simulink model "npc_controller"  (R2022a)
settings: Solver=FixedStepDiscrete  StartTime=0.0  StopTime=20  RelTol=1e-3  EnableMultiTasking=on
undefined symbols (not defined in the file): CAN_O_INT, CANA_BASE, Down, GPTRIP1SEL, GPTRIP2SEL, GPTRIP3SEL, Tsw, TZ1, TZ2, TZ3, Up
libraries: simulink x147, hdlsllib x90, c2802xlib x34, c2837xDlib x20, c280xlib x12, canmsglib x9, c2838xlib x8, idelinklib_common x3, c2806xlib x2, slpidlib x2, c28004xlib x2, c281xlib x2
(part 8 of 42)

== system npc_controller/CONTROL/STATE-MACHINE/CPU_CONTROL_750_A2_precharge_pfc_ok2_OL SS1/disablePwm ==
  note: /*Force PWM to LOW*/
      | EPwm2Regs.AQCSFRC.bit.CSFA = (uint16_T)(0b01);
      | EPwm2Regs.AQCSFRC.bit.CSFB = (uint16_T)(0b01);
      | EPwm7Regs.AQCSFRC.bit.CSFA = (uint16_T)(0b01);
      | EPwm7Regs.AQCSFRC.bit.CSFB = (uint16_T)(0b01);
      | EPwm8Regs.AQCSFRC.bit.CSFA = (uint16_T)(0b01);
      | EPwm8Regs.AQCSFRC.bit.CSFB = (uint16_T)(0b01);
      | EPwm9Regs.AQCSFRC.bit.CSFA = (uint16_T)(0b01);
      | EPwm9Regs.AQCSFRC.bit.CSFB = (uint16_T)(0b01);
      | EPwm10Regs.AQCSFRC.bit.CSFA = (uint16_T)(0b01);
      | EPwm10Regs.AQCSFRC.bit.CSFB = (uint16_T)(0b01);
      | EPwm11Regs.AQCSFRC.bit.CSFA = (uint16_T)(0b01);
      | EPwm11Regs.AQCSFRC.bit.CSFB = (uint16_T)(0b01);
  note: Note:
      | AQCSFRC
      | 0b00 - disables forced PWM
      | 0b01 - forces PWM to LOW
      | 0b10 - forces PWM to  HIGH
  f : TriggerPort  TriggerType=function-call  VariantControl=(inherit)
      settings: CopyFcn=Stateflow.SLINSF.SimulinkMan.removeBlockPreDeleteFcn  PreDeleteFcn=Stateflow.SLINSF.SimulinkMan.unsafePredeleteFcn
  System Outputs : Subsystem  mask(System Outputs){ShowInLibBrowser=0}
      mask prompts: ShowInLibBrowser "Simulink:masks:CustCodeMaskParam1_MP"
      settings: CopyFcn=cccopyfcn(gcb)  OpenFcn=ccopenfcn('System Outputs Function')
      mask Help: eval('feval(''rtwprivate'',''rtwhelpview'',''rtw_sys_outputs_block'')');
      mask Display: disp('System\nOutputs');

== system npc_controller/CONTROL/STATE-MACHINE/CPU_CONTROL_750_A2_precharge_pfc_ok2_OL SS1/enDigCmpMode ==
  note: Note:
      | TZCCTL
      | 0b00 - High impedance
      | 0b01 - Force to HIGH
      | 0b10 - Force to LOW
      | 0b11 - Do nothing
  note: /*Configure TZCTL*/
      | //TZCTL configures TZ action of a DCxEVTy event
      | //0b00=HI-Z, 0b01=HI, 0b10=LO, 0b11=DN
      | EALLOW;
      | EPwm2Regs.TZCTL.bit.DCAEVT1 = 0b10;
      | EPwm2Regs.TZCTL.bit.DCAEVT2 = 0b01;
      | EPwm7Regs.TZCTL.bit.DCAEVT1 = 0b10;
      | EPwm7Regs.TZCTL.bit.DCAEVT2 = 0b01;
      |
      | EPwm8Regs.TZCTL.bit.DCBEVT1 = 0b10;
      | EPwm8Regs.TZCTL.bit.DCBEVT2 = 0b01;
      | EPwm9Regs.TZCTL.bit.DCAEVT1 = 0b10;
      | EPwm9Regs.TZCTL.bit.DCAEVT2 = 0b01;
      |
      | EPwm10Regs.TZCTL.bit.DCBEVT1 = 0b10;
      | EPwm10Regs.TZCTL.bit.DCBEVT2 = 0b01;
      | EPwm11Regs.TZCTL.bit.DCAEVT1 = 0b10;
      | EPwm11Regs.TZCTL.bit.DCAEVT2 = 0b01;
      | EDIS;
  f : TriggerPort  TriggerType=function-call  VariantControl=(inherit)
      settings: CopyFcn=Stateflow.SLINSF.SimulinkMan.removeBlockPreDeleteFcn  PreDeleteFcn=Stateflow.SLINSF.SimulinkMan.unsafePredeleteFcn
  System Outputs2 : Subsystem  mask(System Outputs){ShowInLibBrowser=0}
      mask prompts: ShowInLibBrowser "Simulink:masks:CustCodeMaskParam1_MP"
      settings: CopyFcn=cccopyfcn(gcb)  OpenFcn=ccopenfcn('System Outputs Function')
      mask Help: eval('feval(''rtwprivate'',''rtwhelpview'',''rtw_sys_outputs_block'')');
      mask Display: disp('System\nOutputs');

== system npc_controller/CONTROL/STATE-MACHINE/CPU_CONTROL_750_A2_precharge_pfc_ok2_OL SS1/updateCalib ==
  note: Note: 50 cycles of 50Hz vac
  cnt_calib : Inport  OutDataTypeStr=uint16  PortDimensions=1
  van : Inport  Port=2  OutDataTypeStr=single  PortDimensions=1
  vbn : Inport  Port=3  OutDataTypeStr=single  PortDimensions=1
  vcn : Inport  Port=4  OutDataTypeStr=single  PortDimensions=1
  ia : Inport  Port=5  OutDataTypeStr=single  PortDimensions=1
  ib : Inport  Port=6  OutDataTypeStr=single  PortDimensions=1
  ic : Inport  Port=7  OutDataTypeStr=single  PortDimensions=1
  f : TriggerPort  TriggerType=function-call  VariantControl=(inherit)
      settings: CopyFcn=Stateflow.SLINSF.SimulinkMan.removeBlockPreDeleteFcn  PreDeleteFcn=Stateflow.SLINSF.SimulinkMan.unsafePredeleteFcn
  If : If  IfExpression=u1 > 65000
  If1 : If  Commented=on  IfExpression=u1 > 13000
  Merge : Merge
  Scope : Scope  Commented=on
  cnt : Subsystem  TreatAsAtomicUnit=on
  done : Subsystem  TreatAsAtomicUnit=on
  calib_ok : Outport
  wires:
  cnt_calib/1 -> If/1, cnt/1(cnt_calib)
  cnt/1(calib_ok) -> Merge/2
  done/1(calib_ok) -> Merge/1
  If/1 -> done/Action
  If/2 -> cnt/Action
  Merge/1 -> calib_ok/1, Scope/1
  van/1 -> cnt/2(van)
  vbn/1 -> cnt/3(vbn)
  vcn/1 -> cnt/4(vcn)
  ia/1 -> cnt/5(ia)
  ib/1 -> cnt/6(ib)
  ic/1 -> cnt/7(ic)

== system npc_controller/CONTROL/STATE-MACHINE/CPU_CONTROL_750_A2_precharge_pfc_ok2_OL SS1/updatePll3p ==
  van : Inport  OutDataTypeStr=double  PortDimensions=1
  vbn : Inport  Port=2  OutDataTypeStr=double  PortDimensions=1
  vcn : Inport  Port=3  OutDataTypeStr=double  PortDimensions=1
  f : TriggerPort  TriggerType=function-call  VariantControl=(inherit)
      settings: CopyFcn=Stateflow.SLINSF.SimulinkMan.removeBlockPreDeleteFcn  PreDeleteFcn=Stateflow.SLINSF.SimulinkMan.unsafePredeleteFcn
  Mux : Mux  Inputs=3
  PLL : Subsystem  TreatAsAtomicUnit=on
      settings: RTWFcnNameOpts=Use subsystem name
  Scope : Scope  NumInputPorts=4
  theta : Outport
  wires:
  PLL/1(theta) -> Scope/4, theta/1
  van/1 -> Scope/1, Mux/1
  vcn/1 -> Scope/3, Mux/3
  vbn/1 -> Scope/2, Mux/2
  Mux/1 -> PLL/1(abc)

== system npc_controller/CONTROL/STATE-MACHINE/CPU_CONTROL_750_A2_precharge_pfc_ok2_OL SS1/updateSequencePhA ==
  note: Note:
      | Vmid         C2
      | Vbulk        A5
      |
      | Va            A2/B6
      | Vb            B0
      | Vc            C0
      |
      | Ia             A3
      | Ib             A10/B1, C10
      | Ic             C1
  note: Notes:
      | vac_adc = vac_actual*0.00264706+1.65
      | iac_adc = iac_actual*0.02+1.65
      | vbulk_adc = vbulk_actual*3.49e-3
      | vmid_adc = vmid_acutal*3.49e-3
  vxn : Inport
  ix : Inport  Port=2
  f : TriggerPort  TriggerType=function-call  VariantControl=(inherit)
      settings: CopyFcn=Stateflow.SLINSF.SimulinkMan.removeBlockPreDeleteFcn  PreDeleteFcn=Stateflow.SLINSF.SimulinkMan.unsafePredeleteFcn
  Cast To Single : DataTypeConversion  Commented=on  OutDataTypeStr=single  SaturateOnIntegerOverflow=off  RndMeth=Floor
  Cast To Single1 : DataTypeConversion  Commented=on  OutDataTypeStr=single  SaturateOnIntegerOverflow=off  RndMeth=Floor
  From5 : From  Commented=on  GotoTag=vxn
  From6 : From  Commented=on  GotoTag=pol_vxn
  From7 : From  Commented=on  GotoTag=ix
  From8 : From  Commented=on  GotoTag=pol_ix
  Function-Call Generator : simulink/Ports & Subsystems/Function-Call Generator  sample_time=-1  numberOfIterations=1  DisallowWideOutput=off
  Function-Call Split : FunctionCallSplit  NumOutputPorts=2
  Function-Call Split2 : FunctionCallSplit  NumOutputPorts=2
  Gain2 : Gain  Commented=on  Gain=200
  Gain3 : Gain  Commented=on  Gain=200
  Mux : Mux  Commented=on  Inputs=2
  Mux1 : Mux  Commented=on  Inputs=2
  Scope : Scope  Commented=on  NumInputPorts=3
  pol_final1 : Subsystem  Commented=on
  pol_ix1 : Subsystem  Commented=on
  pol_vxn1 : Subsystem
  vx_seq : Outport
  wires:
  vxn/1 -> [vxn]
  Function-Call Split/2 -> pol_final1/Trigger
  Function-Call Split2/1 -> pol_vxn1/Trigger
  Function-Call Split/1 -> pol_ix1/Trigger
  Function-Call Generator/1 -> Function-Call Split2/1
  Function-Call Split2/2 -> Function-Call Split/1
  [vxn] -> pol_vxn1/1(vxn)
  [ix] -> pol_ix1/1(ix)
  pol_ix1/1(pol_ix) -> [pol_ix]
  [pol_vxn] -> pol_final1/1(vxn)
  [pol_ix] -> pol_final1/2(ix)
  pol_final1/1(pol) -> Scope/3
  Mux/1 -> Scope/1
  Mux1/1 -> Scope/2
  From6/1 -> Cast To Single/1
  From8/1 -> Cast To Single1/1
  Cast To Single/1 -> Gain2/1
  ix/1 -> [ix]
  From5/1 -> Mux/1
  From7/1 -> Mux1/1
  Gain2/1 -> Mux/2
  Cast To Single1/1 -> Gain3/1
  Gain3/1 -> Mux1/2
  [pol_vxn] -> vx_seq/1
  pol_vxn1/1(pol_vxn) -> [pol_vxn]

== system npc_controller/CONTROL/STATE-MACHINE/CPU_CONTROL_750_A2_precharge_pfc_ok2_OL SS1/updateSequencePhB ==
  note: Note:
      | Vmid         C2
      | Vbulk        A5
      |
      | Va            A2/B6
      | Vb            B0
      | Vc            C0
      |
      | Ia             A3
      | Ib             A10/B1, C10
      | Ic             C1
  note: Notes:
      | vac_adc = vac_actual*0.00264706+1.65
      | iac_adc = iac_actual*0.02+1.65
      | vbulk_adc = vbulk_actual*3.49e-3
      | vmid_adc = vmid_acutal*3.49e-3
  note: Note:
      |
      | Function PWM # GPIO # LAUNCHPAD PIN #
      |
      | Synci EPWM1A GPIO0 J4.40
      | EPWM1B GPIO1 J4.39
      |
      | ORPS EPMW2A GPIO2 J4.38
      | EPWM2B GPIO3 J4.37
      |
      | RELAY EPWM3A GPIO4 J4.36
      |
      | TZ GPIO62 XX
      |
      | a_s1 EPWM6A GPIO10 J8.76
      | a_s2 EPWM7B GPIO13 XX
      | a_s3 EPWM6B GPIO11 J8.75
      | a_s4 EPWM7A GPIO12 XX
      |
      | b_s1 EPWM8B GPIO15 J8.73
      | b_s2 EPWM9B GPIO17 XX
      | b_s3 EPWM8A GPIO14 J8.74
      | b_s4 EPWM9A GPIO16 J4.33
      |
      | c_s1 EPWM10B GPIO19 J1.3
      | c_s2 EPWM11B GPIO21 XX
      | c_s3 EPWM10A GPIO18 J1.4
      | c_s4 EPWM11A GPIO20 XX
  vxn : Inport
  ix : Inport  Port=2
  f : TriggerPort  TriggerType=function-call  VariantControl=(inherit)
      settings: CopyFcn=Stateflow.SLINSF.SimulinkMan.removeBlockPreDeleteFcn  PreDeleteFcn=Stateflow.SLINSF.SimulinkMan.unsafePredeleteFcn
  Cast To Single : DataTypeConversion  Commented=on  OutDataTypeStr=single  SaturateOnIntegerOverflow=off  RndMeth=Floor
  Cast To Single1 : DataTypeConversion  Commented=on  OutDataTypeStr=single  SaturateOnIntegerOverflow=off  RndMeth=Floor
  From5 : From  Commented=on  GotoTag=vxn
  From6 : From  Commented=on  GotoTag=pol_vxn
  From7 : From  Commented=on  GotoTag=ix
  From8 : From  Commented=on  GotoTag=pol_ix
  Function-Call Generator : simulink/Ports & Subsystems/Function-Call Generator  sample_time=-1  numberOfIterations=1  DisallowWideOutput=off
  Function-Call Split : FunctionCallSplit  NumOutputPorts=2
  Function-Call Split2 : FunctionCallSplit  NumOutputPorts=2
  Gain2 : Gain  Commented=on  Gain=200
  Gain3 : Gain  Commented=on  Gain=200
  Mux : Mux  Commented=on  Inputs=2
  Mux1 : Mux  Commented=on  Inputs=2
  Scope : Scope  Commented=on  NumInputPorts=3
  pol_final1 : Subsystem  Commented=on
  pol_ix1 : Subsystem  Commented=on
  pol_vxn1 : Subsystem
  vx_seq : Outport
  wires:
  vxn/1 -> [vxn]
  Function-Call Split/2 -> pol_final1/Trigger
  Function-Call Split2/1 -> pol_vxn1/Trigger
  Function-Call Split/1 -> pol_ix1/Trigger
  Function-Call Generator/1 -> Function-Call Split2/1
  Function-Call Split2/2 -> Function-Call Split/1
  [vxn] -> pol_vxn1/1(vxn)
  [ix] -> pol_ix1/1(ix)
  pol_ix1/1(pol_ix) -> [pol_ix]
  [pol_vxn] -> pol_final1/1(vxn)
  [pol_ix] -> pol_final1/2(ix)
  pol_final1/1(pol) -> Scope/3
  Mux/1 -> Scope/1
  Mux1/1 -> Scope/2
  From6/1 -> Cast To Single/1
  From8/1 -> Cast To Single1/1
  Cast To Single/1 -> Gain2/1
  ix/1 -> [ix]
  From5/1 -> Mux/1
  From7/1 -> Mux1/1
  Gain2/1 -> Mux/2
  Cast To Single1/1 -> Gain3/1
  Gain3/1 -> Mux1/2
  [pol_vxn] -> vx_seq/1
  pol_vxn1/1(pol_vxn) -> [pol_vxn]

== system npc_controller/CONTROL/STATE-MACHINE/CPU_CONTROL_750_A2_precharge_pfc_ok2_OL SS1/updateSequencePhC ==
  note: Note:
      | Vmid         C2
      | Vbulk        A5
      |
      | Va            A2/B6
      | Vb            B0
      | Vc            C0
      |
      | Ia             A3
      | Ib             A10/B1, C10
      | Ic             C1
  note: Notes:
      | vac_adc = vac_actual*0.00264706+1.65
      | iac_adc = iac_actual*0.02+1.65
      | vbulk_adc = vbulk_actual*3.49e-3
      | vmid_adc = vmid_acutal*3.49e-3
  note: Note:
      |
      | Function PWM # GPIO # LAUNCHPAD PIN #
      |
      | Synci EPWM1A GPIO0 J4.40
      | EPWM1B GPIO1 J4.39
      |
      | ORPS EPMW2A GPIO2 J4.38
      | EPWM2B GPIO3 J4.37
      |
      | RELAY EPWM3A GPIO4 J4.36
      |
      | TZ GPIO62 XX
      |
      | a_s1 EPWM6A GPIO10 J8.76
      | a_s2 EPWM7B GPIO13 XX
      | a_s3 EPWM6B GPIO11 J8.75
      | a_s4 EPWM7A GPIO12 XX
      |
      | b_s1 EPWM8B GPIO15 J8.73
      | b_s2 EPWM9B GPIO17 XX
      | b_s3 EPWM8A GPIO14 J8.74
      | b_s4 EPWM9A GPIO16 J4.33
      |
      | c_s1 EPWM10B GPIO19 J1.3
      | c_s2 EPWM11B GPIO21 XX
      | c_s3 EPWM10A GPIO18 J1.4
      | c_s4 EPWM11A GPIO20 XX
  vxn : Inport
  ix : Inport  Port=2
  f : TriggerPort  TriggerType=function-call  VariantControl=(inherit)
      settings: CopyFcn=Stateflow.SLINSF.SimulinkMan.removeBlockPreDeleteFcn  PreDeleteFcn=Stateflow.SLINSF.SimulinkMan.unsafePredeleteFcn
  Cast To Single : DataTypeConversion  Commented=on  OutDataTypeStr=single  SaturateOnIntegerOverflow=off  RndMeth=Floor
  Cast To Single1 : DataTypeConversion  Commented=on  OutDataTypeStr=single  SaturateOnIntegerOverflow=off  RndMeth=Floor
  From5 : From  Commented=on  GotoTag=vxn
  From6 : From  Commented=on  GotoTag=pol_vxn
  From7 : From  Commented=on  GotoTag=ix
  From8 : From  Commented=on  GotoTag=pol_ix
  Function-Call Generator : simulink/Ports & Subsystems/Function-Call Generator  sample_time=-1  numberOfIterations=1  DisallowWideOutput=off
  Function-Call Split : FunctionCallSplit  NumOutputPorts=2
  Function-Call Split2 : FunctionCallSplit  NumOutputPorts=2
  Gain2 : Gain  Commented=on  Gain=200
  Gain3 : Gain  Commented=on  Gain=200
  Mux : Mux  Commented=on  Inputs=2
  Mux1 : Mux  Commented=on  Inputs=2
  Scope : Scope  Commented=on  NumInputPorts=3
  pol_final1 : Subsystem  Commented=on
  pol_ix1 : Subsystem  Commented=on
  pol_vxn1 : Subsystem
  vx_seq : Outport
  wires:
  vxn/1 -> [vxn]
  Function-Call Split/2 -> pol_final1/Trigger
  Function-Call Split2/1 -> pol_vxn1/Trigger
  Function-Call Split/1 -> pol_ix1/Trigger
  Function-Call Generator/1 -> Function-Call Split2/1
  Function-Call Split2/2 -> Function-Call Split/1
  [vxn] -> pol_vxn1/1(vxn)
  pol_vxn1/1(pol_vxn) -> [pol_vxn]
  [ix] -> pol_ix1/1(ix)
  pol_ix1/1(pol_ix) -> [pol_ix]
  [pol_vxn] -> pol_final1/1(vxn)
  [pol_ix] -> pol_final1/2(ix)
  pol_final1/1(pol) -> Scope/3
  Mux/1 -> Scope/1
  Mux1/1 -> Scope/2
  From6/1 -> Cast To Single/1
  From8/1 -> Cast To Single1/1
  Cast To Single/1 -> Gain2/1
  ix/1 -> [ix]
  From5/1 -> Mux/1
  From7/1 -> Mux1/1
  Gain2/1 -> Mux/2
  Cast To Single1/1 -> Gain3/1
  Gain3/1 -> Mux1/2
  [pol_vxn] -> vx_seq/1

== system npc_controller/CONTROL/STATE-MACHINE/CPU_CONTROL_750_A2_precharge_pfc_ok2_OL SS2/ClrCmpssTz ==
  note: /*Configure TZCTL*/
      | //TZCTL configures TZ action of a DCxEVTy event
      | //0b00=HI-Z, 0b01=HI, 0b10=LO, 0b11=DN
      | EALLOW;
      | EPwm2Regs.TZCTL.bit.DCAEVT1 = 0b10;
      | EPwm2Regs.TZCTL.bit.DCAEVT2 = 0b01;
      | EPwm7Regs.TZCTL.bit.DCAEVT1 = 0b10;
      | EPwm7Regs.TZCTL.bit.DCAEVT2 = 0b01;
      |
      | EPwm8Regs.TZCTL.bit.DCBEVT1 = 0b10;
      | EPwm8Regs.TZCTL.bit.DCBEVT2 = 0b01;
      | EPwm9Regs.TZCTL.bit.DCAEVT1 = 0b10;
      | EPwm9Regs.TZCTL.bit.DCAEVT2 = 0b01;
      |
      | EPwm10Regs.TZCTL.bit.DCBEVT1 = 0b10;
      | EPwm10Regs.TZCTL.bit.DCBEVT2 = 0b01;
      | EPwm11Regs.TZCTL.bit.DCAEVT1 = 0b10;
      | EPwm11Regs.TZCTL.bit.DCAEVT2 = 0b01;
      | EDIS;
  note: Note:
      | TZCCTL
      | 0b00 - High impedance
      | 0b01 - Force to HIGH
      | 0b10 - Force to LOW
      | 0b11 - Do nothing
  note: /*Configure TZCTL*/
      | //TZCTL configures TZ action of a DCxEVTy event
      | //0b00=HI-Z, 0b01=HI, 0b10=LO, 0b11=DN
      | EALLOW;
      | EPwm2Regs.TZCTL.bit.DCAEVT1 = 0b00;
      | EPwm2Regs.TZCTL.bit.DCBEVT1 = 0b00;
      | EPwm7Regs.TZCTL.bit.DCAEVT1 = 0b00;
      | EPwm7Regs.TZCTL.bit.DCBEVT1 = 0b00;
      |
      | EPwm8Regs.TZCTL.bit.DCAEVT1 = 0b00;
      | EPwm8Regs.TZCTL.bit.DCBEVT1 = 0b00;
      | EPwm9Regs.TZCTL.bit.DCAEVT1 = 0b00;
      | EPwm9Regs.TZCTL.bit.DCBEVT1 = 0b00;
      |
      | EPwm10Regs.TZCTL.bit.DCAEVT1 = 0b00;
      | EPwm10Regs.TZCTL.bit.DCBEVT1 = 0b00;
      | EPwm11Regs.TZCTL.bit.DCAEVT1 = 0b00;
      | EPwm11Regs.TZCTL.bit.DCBEVT1 = 0b00;
      |
      | EDIS;
  f : TriggerPort  TriggerType=function-call  VariantControl=(inherit)
      settings: CopyFcn=Stateflow.SLINSF.SimulinkMan.removeBlockPreDeleteFcn  PreDeleteFcn=Stateflow.SLINSF.SimulinkMan.unsafePredeleteFcn
  System Outputs1 : Subsystem  mask(System Outputs){ShowInLibBrowser=0}
      mask prompts: ShowInLibBrowser "Simulink:masks:CustCodeMaskParam1_MP"
      settings: CopyFcn=cccopyfcn(gcb)  OpenFcn=ccopenfcn('System Outputs Function')
      mask Help: eval('feval(''rtwprivate'',''rtwhelpview'',''rtw_sys_outputs_block'')');
      mask Display: disp('System\nOutputs');
  System Outputs2 : Subsystem  Commented=on  mask(System Outputs){ShowInLibBrowser=0}
      mask prompts: ShowInLibBrowser "Simulink:masks:CustCodeMaskParam1_MP"
      settings: CopyFcn=cccopyfcn(gcb)  OpenFcn=ccopenfcn('System Outputs Function')
      mask Help: eval('feval(''rtwprivate'',''rtwhelpview'',''rtw_sys_outputs_block'')');
      mask Display: disp('System\nOutputs');

== system npc_controller/CONTROL/STATE-MACHINE/CPU_CONTROL_750_A2_precharge_pfc_ok2_OL SS2/configFutDis ==
  note: /*Force PWM to LOW*/
      | EPwm2Regs.AQCSFRC.bit.CSFA = (uint16_T)(0b01); force to LOW
      | EPwm2Regs.AQCSFRC.bit.CSFB = (uint16_T)(0b01);
      | EPwm7Regs.AQCSFRC.bit.CSFA = (uint16_T)(0b01);
      | EPwm7Regs.AQCSFRC.bit.CSFB = (uint16_T)(0b01);
      | EPwm8Regs.AQCSFRC.bit.CSFA = (uint16_T)(0b01);
      | EPwm8Regs.AQCSFRC.bit.CSFB = (uint16_T)(0b01);
      | EPwm9Regs.AQCSFRC.bit.CSFA = (uint16_T)(0b01);
      | EPwm9Regs.AQCSFRC.bit.CSFB = (uint16_T)(0b01);
      | EPwm10Regs.AQCSFRC.bit.CSFA = (uint16_T)(0b01);
      | EPwm10Regs.AQCSFRC.bit.CSFB = (uint16_T)(0b01);
      | EPwm11Regs.AQCSFRC.bit.CSFA = (uint16_T)(0b01);
      | EPwm11Regs.AQCSFRC.bit.CSFB = (uint16_T)(0b01);
  note: /*Force PWM to LOW*/
      | EPwm6Regs.AQCSFRC.bit.CSFA = (uint16_T)(0b01);
      | EPwm6Regs.AQCSFRC.bit.CSFB = (uint16_T)(0b01);
      | EPwm7Regs.AQCSFRC.bit.CSFA = (uint16_T)(0b01);
      | EPwm7Regs.AQCSFRC.bit.CSFB = (uint16_T)(0b01);
      | EPwm8Regs.AQCSFRC.bit.CSFA = (uint16_T)(0b01);
      | EPwm8Regs.AQCSFRC.bit.CSFB = (uint16_T)(0b01);
      | EPwm9Regs.AQCSFRC.bit.CSFA = (uint16_T)(0b01);
      | EPwm9Regs.AQCSFRC.bit.CSFB = (uint16_T)(0b01);
      | EPwm10Regs.AQCSFRC.bit.CSFA = (uint16_T)(0b01);
      | EPwm10Regs.AQCSFRC.bit.CSFB = (uint16_T)(0b01);
      | EPwm11Regs.AQCSFRC.bit.CSFA = (uint16_T)(0b01);
      | EPwm11Regs.AQCSFRC.bit.CSFB = (uint16_T)(0b01);
      |
      | /*Configure TZCTL*/
      | //TZCTL configures TZ action of a DCxEVTy event
      | //0b00=HI-Z, 0b01=HI, 0b10=LO, 0b11=DN
      | EALLOW;
      | EPwm6Regs.TZCTL.bit.DCBEVT1 = 0b10; //LO
      | EPwm6Regs.TZCTL.bit.DCBEVT2 = 0b01; //HI
      | EDIS;
  note: Note:
      | TZCCTL
      | 0b00 - High impedance
      | 0b01 - Force to HIGH
      | 0b10 - Force to LOW
      | 0b11 - Do nothing
      |
      | AQCSFRC
      | 0b00 - disables forced PWM
      | 0b01 - forces PWM to LOW
      | 0b10 - forces PWM to  HIGH
  f : TriggerPort  TriggerType=function-call  VariantControl=(inherit)
      settings: CopyFcn=Stateflow.SLINSF.SimulinkMan.removeBlockPreDeleteFcn  PreDeleteFcn=Stateflow.SLINSF.SimulinkMan.unsafePredeleteFcn
  System Outputs1 : Subsystem  Commented=on  mask(System Outputs){ShowInLibBrowser=0}
      mask prompts: ShowInLibBrowser "Simulink:masks:CustCodeMaskParam1_MP"
      settings: CopyFcn=cccopyfcn(gcb)  OpenFcn=ccopenfcn('System Outputs Function')
      mask Help: eval('feval(''rtwprivate'',''rtwhelpview'',''rtw_sys_outputs_block'')');
      mask Display: disp('System\nOutputs');
  System Outputs2 : Subsystem  mask(System Outputs){ShowInLibBrowser=0}
      mask prompts: ShowInLibBrowser "Simulink:masks:CustCodeMaskParam1_MP"
      settings: CopyFcn=cccopyfcn(gcb)  OpenFcn=ccopenfcn('System Outputs Function')
      mask Help: eval('feval(''rtwprivate'',''rtwhelpview'',''rtw_sys_outputs_block'')');
      mask Display: disp('System\nOutputs');

== system npc_controller/CONTROL/STATE-MACHINE/CPU_CONTROL_750_A2_precharge_pfc_ok2_OL SS2/configFutEn ==
  note: //30%duty bot cap
      | /*Disable forced PWM*/
      | EPwm6Regs.AQCSFRC.bit.CSFB = (uint16_T)(0b10); //HIGH
      | EPwm6Regs.AQCSFRC.bit.CSFA = (uint16_T)(0b01); //LOW
      | EPwm7Regs.AQCSFRC.bit.CSFA = (uint16_T)(0b00);
      | EPwm7Regs.AQCSFRC.bit.CSFB = (uint16_T)(0b00);
      |
      | EPwm8Regs.AQCSFRC.bit.CSFA = (uint16_T)(0b10); //HIGH
      | EPwm8Regs.AQCSFRC.bit.CSFB = (uint16_T)(0b01); //LOW
      | EPwm9Regs.AQCSFRC.bit.CSFA = (uint16_T)(0b00);
      | EPwm9Regs.AQCSFRC.bit.CSFB = (uint16_T)(0b00);
      |
      | EPwm10Regs.AQCSFRC.bit.CSFA = (uint16_T)(0b10); //HIGH
      | EPwm10Regs.AQCSFRC.bit.CSFB = (uint16_T)(0b01); //LOW
      | EPwm11Regs.AQCSFRC.bit.CSFA = (uint16_T)(0b00);
      | EPwm11Regs.AQCSFRC.bit.CSFB = (uint16_T)(0b00);
      |
      | /*Input unique %duty*/
      | EPwm6Regs.CMPB.bit.CMPB = (uint16_T)(461.4F); //S3
      | EPwm6Regs.CMPA.bit.CMPA = (uint16_T)(461.4F); //S1
      | EPwm7Regs.CMPA.bit.CMPA = (uint16_T)(501.4F); //S4
      | EPwm7Regs.CMPB.bit.CMPB = (uint16_T)(421.4F); //S2
      |
      | EPwm8Regs.CMPA.bit.CMPA = (uint16_T)(461.4F); //S3
      | EPwm8Regs.CMPB.bit.CMPB = (uint16_T)(461.4F); //S1
      | EPwm9Regs.CMPA.bit.CMPA = (uint16_T)(501.4F); //S4
      | EPwm9Regs.CMPB.bit.CMPB = (uint16_T)(421.4F); //S2
      |
      | EPwm10Regs.CMPA.bit.CMPA = (uint16_T)(461.4F); //S3
      | EPwm10Regs.CMPB.bit.CMPB = (uint16_T)(461.4F); //S1
      | EPwm11Regs.CMPA.bit.CMPA = (uint16_T)(501.4F); //S4
      | EPwm11Regs.CMPB.bit.CMPB = (uint16_T)(421.4F); //S2
      |
      | /*Configure TZCTL*/
      | //TZCTL configures TZ action of a DCxEVTy event
      | //0b00=HI-Z, 0b01=HI, 0b10=LO, 0b11=DN
      | EALLOW;
      | EPwm6Regs.TZCTL.bit.DCBEVT1 = 0b11;
      | EPwm6Regs.TZCTL.bit.DCBEVT2 = 0b11;
      | EPwm7Regs.TZCTL.bit.DCBEVT1 = 0b11;
      | EPwm7Regs.TZCTL.bit.DCBEVT2 = 0b11;
      |
      | EPwm8Regs.TZCTL.bit.DCBEVT1 = 0b11;
      | EPwm8Regs.TZCTL.bit.DCBEVT2 = 0b11;
      | EPwm9Regs.TZCTL.bit.DCBEVT1 = 0b11;
      | EPwm9Regs.TZCTL.bit.DCBEVT2 = 0b11;
      |
      | EPwm10Regs.TZCTL.bit.DCBEVT1 = 0b11;
      | EPwm10Regs.TZCTL.bit.DCBEVT2 = 0b11;
      | EPwm11Regs.TZCTL.bit.DCBEVT1 = 0b11;
      | EPwm11Regs.TZCTL.bit.DCBEVT2 = 0b11;
      | EDIS;
  note: //30%duty top cap
      | /*Disable forced PWM*/
      | EPwm6Regs.AQCSFRC.bit.CSFB = (uint16_T)(0b00);
      | EPwm6Regs.AQCSFRC.bit.CSFA = (uint16_T)(0b00);
      | EPwm7Regs.AQCSFRC.bit.CSFA = (uint16_T)(0b01); //LOW
      | EPwm7Regs.AQCSFRC.bit.CSFB = (uint16_T)(0b10); //HIGH
      |
      | EPwm8Regs.AQCSFRC.bit.CSFA = (uint16_T)(0b00);
      | EPwm8Regs.AQCSFRC.bit.CSFB = (uint16_T)(0b00);
      | EPwm9Regs.AQCSFRC.bit.CSFA = (uint16_T)(0b01); //LOW
      | EPwm9Regs.AQCSFRC.bit.CSFB = (uint16_T)(0b10); //HIGH
      |
      | EPwm10Regs.AQCSFRC.bit.CSFA = (uint16_T)(0b00);
      | EPwm10Regs.AQCSFRC.bit.CSFB = (uint16_T)(0b00);
      | EPwm11Regs.AQCSFRC.bit.CSFA = (uint16_T)(0b01); //LOW
      | EPwm11Regs.AQCSFRC.bit.CSFB = (uint16_T)(0b10); //HIGH
      |
      | /*Input unique %duty*/
      | EPwm6Regs.CMPB.bit.CMPB = (uint16_T)(421.4F); //S3
      | EPwm6Regs.CMPA.bit.CMPA = (uint16_T)(501.4F); //S1
      | EPwm7Regs.CMPA.bit.CMPA = (uint16_T)(461.4F); //S4
      | EPwm7Regs.CMPB.bit.CMPB = (uint16_T)(461.4F); //S2
      |
      | EPwm8Regs.CMPA.bit.CMPA = (uint16_T)(421.4F); //S3
      | EPwm8Regs.CMPB.bit.CMPB = (uint16_T)(501.4F); //S1
      | EPwm9Regs.CMPA.bit.CMPA = (uint16_T)(461.4F); //S4
      | EPwm9Regs.CMPB.bit.CMPB = (uint16_T)(461.4F); //S2
      |
      | EPwm10Regs.CMPA.bit.CMPA = (uint16_T)(421.4F); //S3
      | EPwm10Regs.CMPB.bit.CMPB = (uint16_T)(501.4F); //S1
      | EPwm11Regs.CMPA.bit.CMPA = (uint16_T)(461.4F); //S4
      | EPwm11Regs.CMPB.bit.CMPB = (uint16_T)(461.4F); //S2
      |
      | /*Configure TZCTL*/
      | //TZCTL configures TZ action of a DCxEVTy event
      | //0b00=HI-Z, 0b01=HI, 0b10=LO, 0b11=DN
      | EALLOW;
      | EPwm6Regs.TZCTL.bit.DCBEVT1 = 0b11;
      | EPwm6Regs.TZCTL.bit.DCBEVT2 = 0b11;
      | EPwm7Regs.TZCTL.bit.DCBEVT1 = 0b11;
      | EPwm7Regs.TZCTL.bit.DCBEVT2 = 0b11;
      |
      | EPwm8Regs.TZCTL.bit.DCBEVT1 = 0b11;
      | EPwm8Regs.TZCTL.bit.DCBEVT2 = 0b11;
      | EPwm9Regs.TZCTL.bit.DCBEVT1 = 0b11;
      | EPwm9Regs.TZCTL.bit.DCBEVT2 = 0b11;
      |
      | EPwm10Regs.TZCTL.bit.DCBEVT1 = 0b11;
      | EPwm10Regs.TZCTL.bit.DCBEVT2 = 0b11;
      | EPwm11Regs.TZCTL.bit.DCBEVT1 = 0b11;
      | EPwm11Regs.TZCTL.bit.DCBEVT2 = 0b11;
      | EDIS;
  note: /*Disable forced PWM*/
      | EPwm2Regs.AQCSFRC.bit.CSFA = (uint16_T)(0b00);
      | EPwm2Regs.AQCSFRC.bit.CSFB = (uint16_T)(0b00);
      | EPwm7Regs.AQCSFRC.bit.CSFA = (uint16_T)(0b00);
      | EPwm7Regs.AQCSFRC.bit.CSFB = (uint16_T)(0b00);
      | EPwm8Regs.AQCSFRC.bit.CSFA = (uint16_T)(0b00);
      | EPwm8Regs.AQCSFRC.bit.CSFB = (uint16_T)(0b00);
      | EPwm9Regs.AQCSFRC.bit.CSFA = (uint16_T)(0b00);
      | EPwm9Regs.AQCSFRC.bit.CSFB = (uint16_T)(0b00);
      | EPwm10Regs.AQCSFRC.bit.CSFA = (uint16_T)(0b00);
      | EPwm10Regs.AQCSFRC.bit.CSFB = (uint16_T)(0b00);
      | EPwm11Regs.AQCSFRC.bit.CSFA = (uint16_T)(0b00);
      | EPwm11Regs.AQCSFRC.bit.CSFB = (uint16_T)(0b00);
      |
      | /*Input unique %duty*/
      | EPwm2Regs.CMPA.bit.CMPA = (uint16_T)(461.4F); //S1
      | EPwm7Regs.CMPB.bit.CMPB = (uint16_T)(461.4F); //S2
      | EPwm2Regs.CMPB.bit.CMPB = (uint16_T)(461.4F); //S3
      | EPwm7Regs.CMPA.bit.CMPA = (uint16_T)(461.4F); //S4
      |
      | EPwm8Regs.CMPB.bit.CMPB = (uint16_T)(922.8F); //S1
      | EPwm9Regs.CMPB.bit.CMPB = (uint16_T)(922.8F); //S2
      | EPwm8Regs.CMPA.bit.CMPA = (uint16_T)(922.8F); //S3
      | EPwm9Regs.CMPA.bit.CMPA = (uint16_T)(922.8F); //S4
      |
      | EPwm10Regs.CMPB.bit.CMPB = (uint16_T)(1384.2F); //S1
      | EPwm11Regs.CMPB.bit.CMPB = (uint16_T)(1384.2F); //S2
      | EPwm10Regs.CMPA.bit.CMPA = (uint16_T)(1384.2F); //S3
      | EPwm11Regs.CMPA.bit.CMPA = (uint16_T)(1384.2F); //S4
  note: Note:
      | TZCCTL
      | 0b00 - High impedance
      | 0b01 - Force to HIGH
      | 0b10 - Force to LOW
      | 0b11 - Do nothing
      |
      | AQCSFRC
      | 0b00 - disables forced PWM
      | 0b01 - forces PWM to LOW
      | 0b10 - forces PWM to  HIGH
  f : TriggerPort  TriggerType=function-call  VariantControl=(inherit)
      settings: CopyFcn=Stateflow.SLINSF.SimulinkMan.removeBlockPreDeleteFcn  PreDeleteFcn=Stateflow.SLINSF.SimulinkMan.unsafePredeleteFcn
  System Outputs1 : Subsystem  mask(System Outputs){ShowInLibBrowser=0}
      mask prompts: ShowInLibBrowser "Simulink:masks:CustCodeMaskParam1_MP"
      settings: CopyFcn=cccopyfcn(gcb)  OpenFcn=ccopenfcn('System Outputs Function')
      mask Help: eval('feval(''rtwprivate'',''rtwhelpview'',''rtw_sys_outputs_block'')');
      mask Display: disp('System\nOutputs');
  System Outputs2 : Subsystem  Commented=on  mask(System Outputs){ShowInLibBrowser=0}
      mask prompts: ShowInLibBrowser "Simulink:masks:CustCodeMaskParam1_MP"
      settings: CopyFcn=cccopyfcn(gcb)  OpenFcn=ccopenfcn('System Outputs Function')
      mask Help: eval('feval(''rtwprivate'',''rtwhelpview'',''rtw_sys_outputs_block'')');
      mask Display: disp('System\nOutputs');
  System Outputs3 : Subsystem  Commented=on  mask(System Outputs){ShowInLibBrowser=0}
      mask prompts: ShowInLibBrowser "Simulink:masks:CustCodeMaskParam1_MP"
      settings: CopyFcn=cccopyfcn(gcb)  OpenFcn=ccopenfcn('System Outputs Function')
      mask Help: eval('feval(''rtwprivate'',''rtwhelpview'',''rtw_sys_outputs_block'')');
      mask Display: disp('System\nOutputs');

== system npc_controller/CONTROL/STATE-MACHINE/CPU_CONTROL_750_A2_precharge_pfc_ok2_OL SS2/configGrid ==
  grid_config : Inport  OutDataTypeStr=double  PortDimensions=1
  sinlgeph_config : Inport  Port=2  OutDataTypeStr=double  PortDimensions=1
  f : TriggerPort  TriggerType=function-call  VariantControl=(inherit)
      settings: CopyFcn=Stateflow.SLINSF.SimulinkMan.removeBlockPreDeleteFcn  PreDeleteFcn=Stateflow.SLINSF.SimulinkMan.unsafePredeleteFcn
  FORCE_TZ : Subsystem
  Function-Call Generator : simulink/Ports & Subsystems/Function-Call Generator  sample_time=-1  numberOfIterations=1  DisallowWideOutput=off
  Function-Call Split1 : FunctionCallSplit  NumOutputPorts=2
  RESET_TZ : Subsystem
  wires:
  sinlgeph_config/1 -> FORCE_TZ/2(sinlgeph_config)
  grid_config/1 -> FORCE_TZ/1(In1)
  Function-Call Generator/1 -> Function-Call Split1/1
  Function-Call Split1/2 -> FORCE_TZ/Trigger
  Function-Call Split1/1 -> RESET_TZ/Trigger

== system npc_controller/CONTROL/STATE-MACHINE/CPU_CONTROL_750_A2_precharge_pfc_ok2_OL SS2/detectUvpOvp ==
  Vpk : Inport
  f : TriggerPort  TriggerType=function-call  VariantControl=(inherit)
      settings: CopyFcn=Stateflow.SLINSF.SimulinkMan.removeBlockPreDeleteFcn  PreDeleteFcn=Stateflow.SLINSF.SimulinkMan.unsafePredeleteFcn
  OR : Logic  Operator=OR  IconShape=distinctive  AllPortsSameDT=off  OutDataTypeStr=boolean
  OVP : Stateflow chart  TreatAsAtomicUnit=on
  UVP : Stateflow chart  TreatAsAtomicUnit=on
  tfv_v_UvpOvp : Outport
  wires:
  Vpk/1 -> OVP/1(Vpk1), UVP/1(Vpk2)
  OR/1 -> tfv_v_UvpOvp/1
  OVP/1(tfv_v_Ovp) -> OR/1
  UVP/1(tfv_v_Uvp) -> OR/2

== system npc_controller/CONTROL/STATE-MACHINE/CPU_CONTROL_750_A2_precharge_pfc_ok2_OL SS2/detectZCPhA ==
  vxn : Inport
  f : TriggerPort  TriggerType=function-call  VariantControl=(inherit)
      settings: CopyFcn=Stateflow.SLINSF.SimulinkMan.removeBlockPreDeleteFcn  PreDeleteFcn=Stateflow.SLINSF.SimulinkMan.unsafePredeleteFcn
  If1 : If  IfExpression="(u1 > -5)  & (u1 < 5)"
  Merge1 : Merge
  false : Subsystem  TreatAsAtomicUnit=on
  true : Subsystem  TreatAsAtomicUnit=on
  phx_en : Outport
  wires:
  vxn/1 -> If1/1
  If1/1 -> true/Action
  false/1(ph_en_out) -> Merge1/2
  If1/2 -> false/Action
  true/1(ph_en) -> Merge1/1
  Merge1/1 -> phx_en/1

== system npc_controller/CONTROL/STATE-MACHINE/CPU_CONTROL_750_A2_precharge_pfc_ok2_OL SS2/detectZCPhB ==
  vxn : Inport
  f : TriggerPort  TriggerType=function-call  VariantControl=(inherit)
      settings: CopyFcn=Stateflow.SLINSF.SimulinkMan.removeBlockPreDeleteFcn  PreDeleteFcn=Stateflow.SLINSF.SimulinkMan.unsafePredeleteFcn
  If1 : If  IfExpression="(u1 > -5)  & (u1 < 5)"
  Merge1 : Merge
  false : Subsystem  TreatAsAtomicUnit=on
  true : Subsystem  TreatAsAtomicUnit=on
  phx_en : Outport
  wires:
  vxn/1 -> If1/1
  If1/1 -> true/Action
  false/1(ph_en_out) -> Merge1/2
  If1/2 -> false/Action
  true/1(ph_en) -> Merge1/1
  Merge1/1 -> phx_en/1

== system npc_controller/CONTROL/STATE-MACHINE/CPU_CONTROL_750_A2_precharge_pfc_ok2_OL SS2/detectZCPhC ==
  vxn : Inport
  f : TriggerPort  TriggerType=function-call  VariantControl=(inherit)
      settings: CopyFcn=Stateflow.SLINSF.SimulinkMan.removeBlockPreDeleteFcn  PreDeleteFcn=Stateflow.SLINSF.SimulinkMan.unsafePredeleteFcn
  If1 : If  IfExpression="(u1 > -5)  & (u1 < 5)"
  Merge1 : Merge
  false : Subsystem  TreatAsAtomicUnit=on
  true : Subsystem  TreatAsAtomicUnit=on
  phx_en : Outport
  wires:
  vxn/1 -> If1/1
  If1/1 -> true/Action
  false/1(ph_en_out) -> Merge1/2
  If1/2 -> false/Action
  true/1(ph_en) -> Merge1/1
  Merge1/1 -> phx_en/1

== system npc_controller/CONTROL/STATE-MACHINE/CPU_CONTROL_750_A2_precharge_pfc_ok2_OL SS2/disCmpssTz ==
  note: /*Configure TZCTL*/
      | //TZCTL configures TZ action of a DCxEVTy event
      | //0b00=HI-Z, 0b01=HI, 0b10=LO, 0b11=DN
      | EALLOW;
      | EPwm2Regs.TZCTL.bit.DCAEVT1 = 0b11;
      | EPwm2Regs.TZCTL.bit.DCAEVT2 = 0b11;
      | EPwm7Regs.TZCTL.bit.DCAEVT1 = 0b11;
      | EPwm7Regs.TZCTL.bit.DCAEVT2 = 0b11;
      |
      | EPwm8Regs.TZCTL.bit.DCBEVT1 = 0b11;
      | EPwm8Regs.TZCTL.bit.DCBEVT2 = 0b11;
      | EPwm9Regs.TZCTL.bit.DCAEVT1 = 0b11;
      | EPwm9Regs.TZCTL.bit.DCAEVT2 = 0b11;
      |
      | EPwm10Regs.TZCTL.bit.DCBEVT1 = 0b11;
      | EPwm10Regs.TZCTL.bit.DCBEVT2 = 0b11;
      | EPwm11Regs.TZCTL.bit.DCAEVT1 = 0b11;
      | EPwm11Regs.TZCTL.bit.DCAEVT2 = 0b11;
      | EDIS;
  note: Note:
      | TZCCTL
      | 0b00 - High impedance
      | 0b01 - Force to HIGH
      | 0b10 - Force to LOW
      | 0b11 - Do nothing
  note: /*Configure TZCTL*/
      | //TZCTL configures TZ action of a DCxEVTy event
      | //0b00=HI-Z, 0b01=HI, 0b10=LO, 0b11=DN
      | EALLOW;
      | EPwm2Regs.TZCTL.bit.DCAEVT1 = 0b11;
      | EPwm2Regs.TZCTL.bit.DCBEVT1 = 0b11;
      | EPwm7Regs.TZCTL.bit.DCAEVT1 = 0b11;
      | EPwm7Regs.TZCTL.bit.DCBEVT1 = 0b11;
      |
      | EPwm8Regs.TZCTL.bit.DCAEVT1 = 0b11;
      | EPwm8Regs.TZCTL.bit.DCBEVT1 = 0b11;
      | EPwm9Regs.TZCTL.bit.DCAEVT1 = 0b11;
      | EPwm9Regs.TZCTL.bit.DCBEVT1 = 0b11;
      |
      | EPwm10Regs.TZCTL.bit.DCAEVT1 = 0b11;
      | EPwm10Regs.TZCTL.bit.DCBEVT1 = 0b11;
      | EPwm11Regs.TZCTL.bit.DCAEVT1 = 0b11;
      | EPwm11Regs.TZCTL.bit.DCBEVT1 = 0b11;
      | EDIS;
  f : TriggerPort  TriggerType=function-call  VariantControl=(inherit)
      settings: CopyFcn=Stateflow.SLINSF.SimulinkMan.removeBlockPreDeleteFcn  PreDeleteFcn=Stateflow.SLINSF.SimulinkMan.unsafePredeleteFcn
  System Outputs1 : Subsystem  mask(System Outputs){ShowInLibBrowser=0}
      mask prompts: ShowInLibBrowser "Simulink:masks:CustCodeMaskParam1_MP"
      settings: CopyFcn=cccopyfcn(gcb)  OpenFcn=ccopenfcn('System Outputs Function')
      mask Help: eval('feval(''rtwprivate'',''rtwhelpview'',''rtw_sys_outputs_block'')');
      mask Display: disp('System\nOutputs');
  System Outputs2 : Subsystem  Commented=on  mask(System Outputs){ShowInLibBrowser=0}
      mask prompts: ShowInLibBrowser "Simulink:masks:CustCodeMaskParam1_MP"
      settings: CopyFcn=cccopyfcn(gcb)  OpenFcn=ccopenfcn('System Outputs Function')
      mask Help: eval('feval(''rtwprivate'',''rtwhelpview'',''rtw_sys_outputs_block'')');
      mask Display: disp('System\nOutputs');

== system npc_controller/CONTROL/STATE-MACHINE/CPU_CONTROL_750_A2_precharge_pfc_ok2_OL SS2/disablePwm ==
  note: Note:
      | AQCSFRC
      | 0b00 - disables forced PWM
      | 0b01 - forces PWM to LOW
      | 0b10 - forces PWM to  HIGH
  note: /*Force PWM to LOW*/
      | EPwm2Regs.AQCSFRC.bit.CSFA = (uint16_T)(0b01);
      | EPwm2Regs.AQCSFRC.bit.CSFB = (uint16_T)(0b01);
      | EPwm7Regs.AQCSFRC.bit.CSFA = (uint16_T)(0b01);
      | EPwm7Regs.AQCSFRC.bit.CSFB = (uint16_T)(0b01);
      | EPwm8Regs.AQCSFRC.bit.CSFA = (uint16_T)(0b01);
      | EPwm8Regs.AQCSFRC.bit.CSFB = (uint16_T)(0b01);
      | EPwm9Regs.AQCSFRC.bit.CSFA = (uint16_T)(0b01);
      | EPwm9Regs.AQCSFRC.bit.CSFB = (uint16_T)(0b01);
      | EPwm10Regs.AQCSFRC.bit.CSFA = (uint16_T)(0b01);
      | EPwm10Regs.AQCSFRC.bit.CSFB = (uint16_T)(0b01);
      | EPwm11Regs.AQCSFRC.bit.CSFA = (uint16_T)(0b01);
      | EPwm11Regs.AQCSFRC.bit.CSFB = (uint16_T)(0b01);
  f : TriggerPort  TriggerType=function-call  VariantControl=(inherit)
      settings: CopyFcn=Stateflow.SLINSF.SimulinkMan.removeBlockPreDeleteFcn  PreDeleteFcn=Stateflow.SLINSF.SimulinkMan.unsafePredeleteFcn
  System Outputs : Subsystem  mask(System Outputs){ShowInLibBrowser=0}
      mask prompts: ShowInLibBrowser "Simulink:masks:CustCodeMaskParam1_MP"
      settings: CopyFcn=cccopyfcn(gcb)  OpenFcn=ccopenfcn('System Outputs Function')
      mask Help: eval('feval(''rtwprivate'',''rtwhelpview'',''rtw_sys_outputs_block'')');
      mask Display: disp('System\nOutputs');

== system npc_controller/CONTROL/STATE-MACHINE/CPU_CONTROL_750_A2_precharge_pfc_ok2_OL SS2/readCmpssOcp ==
  note: /*read Digital Compare EVT1 Tz Flag*/
      | npc_controller_DWork .tz_cmpssocp = EPwm2Regs.TZFLG.bit.DCAEVT1 | EPwm2Regs.TZFLG.bit.DCBEVT1 | EPwm7Regs.TZFLG.bit.DCAEVT1 | EPwm7Regs.TZFLG.bit.DCBEVT1 | EPwm8Regs.TZFLG.bit.DCAEVT1 | EPwm8Regs.TZFLG.bit.DCBEVT1 | EPwm9Regs.TZFLG.bit.DCAEVT1 | EPwm9Regs.TZFLG.bit.DCBEVT1| EPwm10Regs.TZFLG.bit.DCAEVT1 | EPwm10Regs.TZFLG.bit.DCBEVT1 | EPwm11Regs.TZFLG.bit.DCAEVT1 | EPwm11Regs.TZFLG.bit.DCBEVT1;
  f : TriggerPort  TriggerType=function-call  VariantControl=(inherit)
      settings: CopyFcn=Stateflow.SLINSF.SimulinkMan.removeBlockPreDeleteFcn  PreDeleteFcn=Stateflow.SLINSF.SimulinkMan.unsafePredeleteFcn
  System Outputs1 : Subsystem  mask(System Outputs){ShowInLibBrowser=0}
      mask prompts: ShowInLibBrowser "Simulink:masks:CustCodeMaskParam1_MP"
      settings: CopyFcn=cccopyfcn(gcb)  OpenFcn=ccopenfcn('System Outputs Function')
      mask Help: eval('feval(''rtwprivate'',''rtwhelpview'',''rtw_sys_outputs_block'')');
      mask Display: disp('System\nOutputs');

== system npc_controller/CONTROL/STATE-MACHINE/CPU_CONTROL_750_A2_precharge_pfc_ok2_OL SS2/updateCalib ==
  note: Note: 50 cycles of 50Hz vac
  cnt_calib : Inport  OutDataTypeStr=uint16  PortDimensions=1
  van : Inport  Port=2  OutDataTypeStr=single  PortDimensions=1
  vbn : Inport  Port=3  OutDataTypeStr=single  PortDimensions=1
  vcn : Inport  Port=4  OutDataTypeStr=single  PortDimensions=1
  ia : Inport  Port=5  OutDataTypeStr=single  PortDimensions=1
  ib : Inport  Port=6  OutDataTypeStr=single  PortDimensions=1
  ic : Inport  Port=7  OutDataTypeStr=single  PortDimensions=1
  f : TriggerPort  TriggerType=function-call  VariantControl=(inherit)
      settings: CopyFcn=Stateflow.SLINSF.SimulinkMan.removeBlockPreDeleteFcn  PreDeleteFcn=Stateflow.SLINSF.SimulinkMan.unsafePredeleteFcn
  If : If  IfExpression=u1 > 6500
  If1 : If  Commented=on  IfExpression=u1 > 13000
  Merge : Merge
  Scope : Scope  Commented=on
  cnt : Subsystem  TreatAsAtomicUnit=on
  done : Subsystem  TreatAsAtomicUnit=on
  calib_ok : Outport
  wires:
  ic/1 -> cnt/7(ic)
  ib/1 -> cnt/6(ib)
  ia/1 -> cnt/5(ia)
  vcn/1 -> cnt/4(vcn)
  vbn/1 -> cnt/3(vbn)
  van/1 -> cnt/2(van)
  Merge/1 -> Scope/1, calib_ok/1
  If/2 -> cnt/Action
  If/1 -> done/Action
  done/1(calib_ok) -> Merge/1
  cnt/1(calib_ok) -> Merge/2
  cnt_calib/1 -> cnt/1(cnt_calib), If/1

== system npc_controller/CONTROL/STATE-MACHINE/CPU_CONTROL_750_A2_precharge_pfc_ok2_OL SS2/updatePll3p ==
  van : Inport  OutDataTypeStr=double  PortDimensions=1
  vbn : Inport  Port=2  OutDataTypeStr=double  PortDimensions=1
  vcn : Inport  Port=3  OutDataTypeStr=double  PortDimensions=1
  f : TriggerPort  TriggerType=function-call  VariantControl=(inherit)
      settings: CopyFcn=Stateflow.SLINSF.SimulinkMan.removeBlockPreDeleteFcn  PreDeleteFcn=Stateflow.SLINSF.SimulinkMan.unsafePredeleteFcn
  Mux : Mux  Inputs=3
  PLL : Subsystem  TreatAsAtomicUnit=on
      settings: RTWFcnNameOpts=Use subsystem name
  Scope : Scope  NumInputPorts=4
  theta : Outport
  wires:
  Mux/1 -> PLL/1(abc)
  vbn/1 -> Mux/2, Scope/2
  vcn/1 -> Mux/3, Scope/3
  van/1 -> Mux/1, Scope/1
  PLL/1(theta) -> theta/1, Scope/4

== system npc_controller/CONTROL/STATE-MACHINE/CPU_CONTROL_750_A2_precharge_pfc_ok2_OL SS2/updateSequencePhA ==
  note: Notes:
      | vac_adc = vac_actual*0.00264706+1.65
      | iac_adc = iac_actual*0.02+1.65
      | vbulk_adc = vbulk_actual*3.49e-3
      | vmid_adc = vmid_acutal*3.49e-3
  note: Note:
      | Vmid         C2
      | Vbulk        A5
      |
      | Va            A2/B6
      | Vb            B0
      | Vc            C0
      |
      | Ia             A3
      | Ib             A10/B1, C10
      | Ic             C1
  vxn : Inport
  ix : Inport  Port=2
  f : TriggerPort  TriggerType=function-call  VariantControl=(inherit)
      settings: CopyFcn=Stateflow.SLINSF.SimulinkMan.removeBlockPreDeleteFcn  PreDeleteFcn=Stateflow.SLINSF.SimulinkMan.unsafePredeleteFcn
  Cast To Single : DataTypeConversion  Commented=on  OutDataTypeStr=single  SaturateOnIntegerOverflow=off  RndMeth=Floor
  Cast To Single1 : DataTypeConversion  Commented=on  OutDataTypeStr=single  SaturateOnIntegerOverflow=off  RndMeth=Floor
  From5 : From  Commented=on  GotoTag=vxn
  From6 : From  Commented=on  GotoTag=pol_vxn
  From7 : From  Commented=on  GotoTag=ix
  From8 : From  Commented=on  GotoTag=pol_ix
  Function-Call Generator : simulink/Ports & Subsystems/Function-Call Generator  sample_time=-1  numberOfIterations=1  DisallowWideOutput=off
  Function-Call Split : FunctionCallSplit  NumOutputPorts=2
  Function-Call Split2 : FunctionCallSplit  NumOutputPorts=2
  Gain2 : Gain  Commented=on  Gain=200
  Gain3 : Gain  Commented=on  Gain=200
  Mux : Mux  Commented=on  Inputs=2
  Mux1 : Mux  Commented=on  Inputs=2
  Scope : Scope  Commented=on  NumInputPorts=3
  pol_final1 : Subsystem  Commented=on
  pol_ix1 : Subsystem  Commented=on
  pol_vxn1 : Subsystem
  pol_vxn2 : Subsystem  Commented=on
  vx_seq : Outport
  wires:
  pol_vxn1/1(pol_vxn) -> [pol_vxn]
  [pol_vxn] -> vx_seq/1
  Gain3/1 -> Mux1/2
  Cast To Single1/1 -> Gain3/1
  Gain2/1 -> Mux/2
  From7/1 -> Mux1/1
  From5/1 -> Mux/1
  ix/1 -> [ix]
  Cast To Single/1 -> Gain2/1
  From8/1 -> Cast To Single1/1
  From6/1 -> Cast To Single/1
  Mux1/1 -> Scope/2
  Mux/1 -> Scope/1
  pol_final1/1(pol) -> Scope/3
  [pol_ix] -> pol_final1/2(ix)
  [pol_vxn] -> pol_final1/1(vxn)
  pol_ix1/1(pol_ix) -> [pol_ix]
  [ix] -> pol_ix1/1(ix)
  [vxn] -> pol_vxn1/1(vxn)
  Function-Call Split2/2 -> Function-Call Split/1
  Function-Call Generator/1 -> Function-Call Split2/1
  Function-Call Split/1 -> pol_ix1/Trigger
  Function-Call Split2/1 -> pol_vxn1/Trigger
  Function-Call Split/2 -> pol_final1/Trigger
  vxn/1 -> [vxn]
  [ix] -> pol_vxn1/2(ixn1)

== system npc_controller/CONTROL/STATE-MACHINE/CPU_CONTROL_750_A2_precharge_pfc_ok2_OL SS2/updateSequencePhB ==
  note: Note:
      |
      | Function PWM # GPIO # LAUNCHPAD PIN #
      |
      | Synci EPWM1A GPIO0 J4.40
      | EPWM1B GPIO1 J4.39
      |
      | ORPS EPMW2A GPIO2 J4.38
      | EPWM2B GPIO3 J4.37
      |
      | RELAY EPWM3A GPIO4 J4.36
      |
      | TZ GPIO62 XX
      |
      | a_s1 EPWM6A GPIO10 J8.76
      | a_s2 EPWM7B GPIO13 XX
      | a_s3 EPWM6B GPIO11 J8.75
      | a_s4 EPWM7A GPIO12 XX
      |
      | b_s1 EPWM8B GPIO15 J8.73
      | b_s2 EPWM9B GPIO17 XX
      | b_s3 EPWM8A GPIO14 J8.74
      | b_s4 EPWM9A GPIO16 J4.33
      |
      | c_s1 EPWM10B GPIO19 J1.3
      | c_s2 EPWM11B GPIO21 XX
      | c_s3 EPWM10A GPIO18 J1.4
      | c_s4 EPWM11A GPIO20 XX
  note: Notes:
      | vac_adc = vac_actual*0.00264706+1.65
      | iac_adc = iac_actual*0.02+1.65
      | vbulk_adc = vbulk_actual*3.49e-3
      | vmid_adc = vmid_acutal*3.49e-3
  note: Note:
      | Vmid         C2
      | Vbulk        A5
      |
      | Va            A2/B6
      | Vb            B0
      | Vc            C0
      |
      | Ia             A3
      | Ib             A10/B1, C10
      | Ic             C1
  vxn : Inport
  ix : Inport  Port=2
  f : TriggerPort  TriggerType=function-call  VariantControl=(inherit)
      settings: CopyFcn=Stateflow.SLINSF.SimulinkMan.removeBlockPreDeleteFcn  PreDeleteFcn=Stateflow.SLINSF.SimulinkMan.unsafePredeleteFcn
  Cast To Single : DataTypeConversion  Commented=on  OutDataTypeStr=single  SaturateOnIntegerOverflow=off  RndMeth=Floor
  Cast To Single1 : DataTypeConversion  Commented=on  OutDataTypeStr=single  SaturateOnIntegerOverflow=off  RndMeth=Floor
  From5 : From  Commented=on  GotoTag=vxn
  From6 : From  Commented=on  GotoTag=pol_vxn
  From7 : From  Commented=on  GotoTag=ix
  From8 : From  Commented=on  GotoTag=pol_ix
  Function-Call Generator : simulink/Ports & Subsystems/Function-Call Generator  sample_time=-1  numberOfIterations=1  DisallowWideOutput=off
  Function-Call Split : FunctionCallSplit  NumOutputPorts=2
  Function-Call Split2 : FunctionCallSplit  NumOutputPorts=2
  Gain2 : Gain  Commented=on  Gain=200
  Gain3 : Gain  Commented=on  Gain=200
  Mux : Mux  Commented=on  Inputs=2
  Mux1 : Mux  Commented=on  Inputs=2
  Scope : Scope  Commented=on  NumInputPorts=3
  pol_final1 : Subsystem  Commented=on
  pol_ix1 : Subsystem  Commented=on
  pol_vxn1 : Subsystem
  pol_vxn2 : Subsystem  Commented=on
  vx_seq : Outport
  wires:
  pol_vxn1/1(pol_vxn) -> [pol_vxn]
  [pol_vxn] -> vx_seq/1
  Gain3/1 -> Mux1/2
  Cast To Single1/1 -> Gain3/1
  Gain2/1 -> Mux/2
  From7/1 -> Mux1/1
  From5/1 -> Mux/1
  ix/1 -> [ix]
  Cast To Single/1 -> Gain2/1
  From8/1 -> Cast To Single1/1
  From6/1 -> Cast To Single/1
  Mux1/1 -> Scope/2
  Mux/1 -> Scope/1
  pol_final1/1(pol) -> Scope/3
  [pol_ix] -> pol_final1/2(ix)
  [pol_vxn] -> pol_final1/1(vxn)
  pol_ix1/1(pol_ix) -> [pol_ix]
  [ix] -> pol_ix1/1(ix)
  [vxn] -> pol_vxn1/1(vxn)
  Function-Call Split2/2 -> Function-Call Split/1
  Function-Call Generator/1 -> Function-Call Split2/1
  Function-Call Split/1 -> pol_ix1/Trigger
  Function-Call Split2/1 -> pol_vxn1/Trigger
  Function-Call Split/2 -> pol_final1/Trigger
  vxn/1 -> [vxn]
  [ix] -> pol_vxn1/2(ixn1)

== system npc_controller/CONTROL/STATE-MACHINE/CPU_CONTROL_750_A2_precharge_pfc_ok2_OL SS2/updateSequencePhC ==
  note: Note:
      |
      | Function PWM # GPIO # LAUNCHPAD PIN #
      |
      | Synci EPWM1A GPIO0 J4.40
      | EPWM1B GPIO1 J4.39
      |
      | ORPS EPMW2A GPIO2 J4.38
      | EPWM2B GPIO3 J4.37
      |
      | RELAY EPWM3A GPIO4 J4.36
      |
      | TZ GPIO62 XX
      |
      | a_s1 EPWM6A GPIO10 J8.76
      | a_s2 EPWM7B GPIO13 XX
      | a_s3 EPWM6B GPIO11 J8.75
      | a_s4 EPWM7A GPIO12 XX
      |
      | b_s1 EPWM8B GPIO15 J8.73
      | b_s2 EPWM9B GPIO17 XX
      | b_s3 EPWM8A GPIO14 J8.74
      | b_s4 EPWM9A GPIO16 J4.33
      |
      | c_s1 EPWM10B GPIO19 J1.3
      | c_s2 EPWM11B GPIO21 XX
      | c_s3 EPWM10A GPIO18 J1.4
      | c_s4 EPWM11A GPIO20 XX
  note: Notes:
      | vac_adc = vac_actual*0.00264706+1.65
      | iac_adc = iac_actual*0.02+1.65
      | vbulk_adc = vbulk_actual*3.49e-3
      | vmid_adc = vmid_acutal*3.49e-3
  note: Note:
      | Vmid         C2
      | Vbulk        A5
      |
      | Va            A2/B6
      | Vb            B0
      | Vc            C0
      |
      | Ia             A3
      | Ib             A10/B1, C10
      | Ic             C1
  vxn : Inport
  ix : Inport  Port=2
  f : TriggerPort  TriggerType=function-call  VariantControl=(inherit)
      settings: CopyFcn=Stateflow.SLINSF.SimulinkMan.removeBlockPreDeleteFcn  PreDeleteFcn=Stateflow.SLINSF.SimulinkMan.unsafePredeleteFcn
  Cast To Single : DataTypeConversion  Commented=on  OutDataTypeStr=single  SaturateOnIntegerOverflow=off  RndMeth=Floor
  Cast To Single1 : DataTypeConversion  Commented=on  OutDataTypeStr=single  SaturateOnIntegerOverflow=off  RndMeth=Floor
  From5 : From  Commented=on  GotoTag=vxn
  From6 : From  Commented=on  GotoTag=pol_vxn
  From7 : From  Commented=on  GotoTag=ix
  From8 : From  Commented=on  GotoTag=pol_ix
  Function-Call Generator : simulink/Ports & Subsystems/Function-Call Generator  sample_time=-1  numberOfIterations=1  DisallowWideOutput=off
  Function-Call Split : FunctionCallSplit  NumOutputPorts=2
  Function-Call Split2 : FunctionCallSplit  NumOutputPorts=2
  Gain2 : Gain  Commented=on  Gain=200
  Gain3 : Gain  Commented=on  Gain=200
  Mux : Mux  Commented=on  Inputs=2
  Mux1 : Mux  Commented=on  Inputs=2
  Scope : Scope  Commented=on  NumInputPorts=3
  pol_final1 : Subsystem  Commented=on
  pol_ix1 : Subsystem  Commented=on
  pol_vxn1 : Subsystem
  pol_vxn2 : Subsystem  Commented=on
  vx_seq : Outport
  wires:
  [pol_vxn] -> vx_seq/1
  Gain3/1 -> Mux1/2
  Cast To Single1/1 -> Gain3/1
  Gain2/1 -> Mux/2
  From7/1 -> Mux1/1
  From5/1 -> Mux/1
  ix/1 -> [ix]
  Cast To Single/1 -> Gain2/1
  From8/1 -> Cast To Single1/1
  From6/1 -> Cast To Single/1
  Mux1/1 -> Scope/2
  Mux/1 -> Scope/1
  pol_final1/1(pol) -> Scope/3
  [pol_ix] -> pol_final1/2(ix)
  [pol_vxn] -> pol_final1/1(vxn)
  pol_ix1/1(pol_ix) -> [pol_ix]
  [ix] -> pol_ix1/1(ix)
  pol_vxn1/1(pol_vxn) -> [pol_vxn]
  [vxn] -> pol_vxn1/1(vxn)
  Function-Call Split2/2 -> Function-Call Split/1
  Function-Call Generator/1 -> Function-Call Split2/1
  Function-Call Split/1 -> pol_ix1/Trigger
  Function-Call Split2/1 -> pol_vxn1/Trigger
  Function-Call Split/2 -> pol_final1/Trigger
  vxn/1 -> [vxn]
  [ix] -> pol_vxn1/2(ixn)

== system npc_controller/CONTROL/STATE-MACHINE/CPU_CONTROL_750_Vpk/configFutDis ==
  note: Note:
      | TZCCTL
      | 0b00 - High impedance
      | 0b01 - Force to HIGH
      | 0b10 - Force to LOW
      | 0b11 - Do nothing
      |
      | AQCSFRC
      | 0b00 - disables forced PWM
      | 0b01 - forces PWM to LOW
      | 0b10 - forces PWM to  HIGH
  note: /*Force PWM to LOW*/
      | EPwm6Regs.AQCSFRC.bit.CSFA = (uint16_T)(0b01);
      | EPwm6Regs.AQCSFRC.bit.CSFB = (uint16_T)(0b01);
      | EPwm7Regs.AQCSFRC.bit.CSFA = (uint16_T)(0b01);
      | EPwm7Regs.AQCSFRC.bit.CSFB = (uint16_T)(0b01);
      | EPwm8Regs.AQCSFRC.bit.CSFA = (uint16_T)(0b01);
      | EPwm8Regs.AQCSFRC.bit.CSFB = (uint16_T)(0b01);
      | EPwm9Regs.AQCSFRC.bit.CSFA = (uint16_T)(0b01);
      | EPwm9Regs.AQCSFRC.bit.CSFB = (uint16_T)(0b01);
      | EPwm10Regs.AQCSFRC.bit.CSFA = (uint16_T)(0b01);
      | EPwm10Regs.AQCSFRC.bit.CSFB = (uint16_T)(0b01);
      | EPwm11Regs.AQCSFRC.bit.CSFA = (uint16_T)(0b01);
      | EPwm11Regs.AQCSFRC.bit.CSFB = (uint16_T)(0b01);
      |
      | /*Configure TZCTL*/
      | //TZCTL configures TZ action of a DCxEVTy event
      | //0b00=HI-Z, 0b01=HI, 0b10=LO, 0b11=DN
      | EALLOW;
      | EPwm6Regs.TZCTL.bit.DCBEVT1 = 0b10; //LO
      | EPwm6Regs.TZCTL.bit.DCBEVT2 = 0b01; //HI
      | EDIS;
  note: /*Force PWM to LOW*/
      | EPwm6Regs.AQCSFRC.bit.CSFA = (uint16_T)(0b01); force to LOW
      | EPwm6Regs.AQCSFRC.bit.CSFB = (uint16_T)(0b01);
      | EPwm7Regs.AQCSFRC.bit.CSFA = (uint16_T)(0b01);
      | EPwm7Regs.AQCSFRC.bit.CSFB = (uint16_T)(0b01);
      | EPwm8Regs.AQCSFRC.bit.CSFA = (uint16_T)(0b01);
      | EPwm8Regs.AQCSFRC.bit.CSFB = (uint16_T)(0b01);
      | EPwm9Regs.AQCSFRC.bit.CSFA = (uint16_T)(0b01);
      | EPwm9Regs.AQCSFRC.bit.CSFB = (uint16_T)(0b01);
      | EPwm10Regs.AQCSFRC.bit.CSFA = (uint16_T)(0b01);
      | EPwm10Regs.AQCSFRC.bit.CSFB = (uint16_T)(0b01);
      | EPwm11Regs.AQCSFRC.bit.CSFA = (uint16_T)(0b01);
      | EPwm11Regs.AQCSFRC.bit.CSFB = (uint16_T)(0b01);
  note: Note:
      |
      | Function PWM # GPIO # LAUNCHPAD PIN #
      |
      | Synci EPWM1A GPIO0 J4.40
      | EPWM1B GPIO1 J4.39
      |
      | ORPS EPMW2A GPIO2 J4.38
      | EPWM2B GPIO3 J4.37
      |
      | RELAY EPWM3A GPIO4 J4.36
      |
      | TZ GPIO62 XX
      |
      | a_s1 EPWM6A GPIO10 J8.76
      | a_s2 EPWM7B GPIO13 XX
      | a_s3 EPWM6B GPIO11 J8.75
      | a_s4 EPWM7A GPIO12 XX
      |
      | b_s1 EPWM8B GPIO15 J8.73
      | b_s2 EPWM9B GPIO17 XX
      | b_s3 EPWM8A GPIO14 J8.74
      | b_s4 EPWM9A GPIO16 J4.33
      |
      | c_s1 EPWM10B GPIO19 J1.3
      | c_s2 EPWM11B GPIO21 XX
      | c_s3 EPWM10A GPIO18 J1.4
      | c_s4 EPWM11A GPIO20 XX
  f : TriggerPort  TriggerType=function-call  VariantControl=(inherit)
      settings: CopyFcn=Stateflow.SLINSF.SimulinkMan.removeBlockPreDeleteFcn  PreDeleteFcn=Stateflow.SLINSF.SimulinkMan.unsafePredeleteFcn
  System Outputs1 : Subsystem  Commented=on  mask(System Outputs){ShowInLibBrowser=0}
      mask prompts: ShowInLibBrowser "Simulink:masks:CustCodeMaskParam1_MP"
      settings: CopyFcn=cccopyfcn(gcb)  OpenFcn=ccopenfcn('System Outputs Function')
      mask Help: eval('feval(''rtwprivate'',''rtwhelpview'',''rtw_sys_outputs_block'')');
      mask Display: disp('System\nOutputs');
  System Outputs2 : Subsystem  mask(System Outputs){ShowInLibBrowser=0}
      mask prompts: ShowInLibBrowser "Simulink:masks:CustCodeMaskParam1_MP"
      settings: CopyFcn=cccopyfcn(gcb)  OpenFcn=ccopenfcn('System Outputs Function')
      mask Help: eval('feval(''rtwprivate'',''rtwhelpview'',''rtw_sys_outputs_block'')');
      mask Display: disp('System\nOutputs');
